simulink model "ResampleoV_I_SOC_16"  (R2016a)
settings: Solver=FixedStepAuto  SolverMode=SingleTasking  StartTime=0.0  StopTime=10000  FixedStep=0.1  RelTol=1e-3
settings Model: Creator=Martin  LastModifiedBy=Martin
settings DebuggingCC: SFUnexpectedBacktrackingDiag=error  SFNoUnconditionalDefaultTransitionDiag=error
settings GRTTargetCC: TargetLangStandard=C99 (ISO)  GeneratePreprocessorConditionals=Use local settings
settings ConfigComp: CovMetricSettings=dwe  CovHtmlReporting=off  CovSaveCumulativeToWorkspaceVar=off  CovSaveSingleToWorkspaceVar=off  CovExternalEMLEnable=on

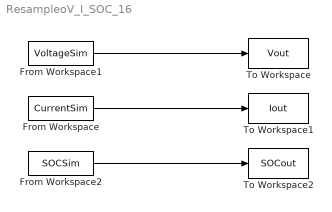
== system ResampleoV_I_SOC_16 ==
  From Workspace : FromWorkspace  VariableName=CurrentSim  SampleTime=0
  From Workspace1 : FromWorkspace  VariableName=VoltageSim  SampleTime=0
  From Workspace2 : FromWorkspace  VariableName=SOCSim  SampleTime=0
  To Workspace : ToWorkspace  VariableName=Vout  SaveFormat=Timeseries  SampleTime=-1
  To Workspace1 : ToWorkspace  VariableName=Iout  SaveFormat=Timeseries  SampleTime=-1
  To Workspace2 : ToWorkspace  VariableName=SOCout  SaveFormat=Timeseries  SampleTime=-1
  wires:
  From Workspace2/1 -> To Workspace2/1
  From Workspace/1 -> To Workspace1/1
  From Workspace1/1 -> To Workspace/1
